simulink model "Utkarsh_2005574_R_W1_P3"  (R2021a)
settings: Solver=FixedStepDiscrete  StartTime=0.0  StopTime=0.1  RelTol=1e-3
settings Model: Creator=Utkarsh Anand  LastModifiedBy=Utkarsh Anand

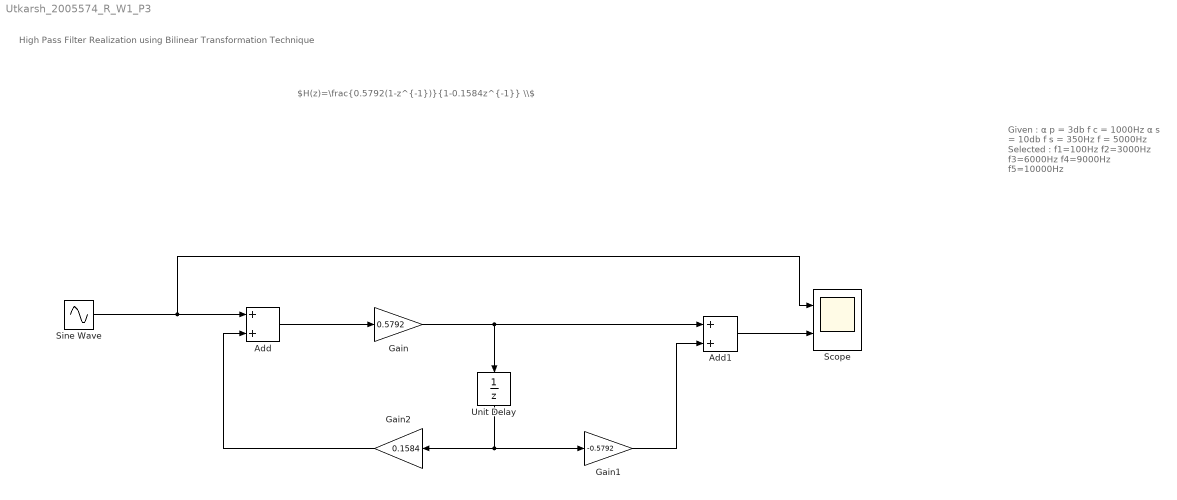
== system Utkarsh_2005574_R_W1_P3 ==
  note: $H(z)=\frac{0.5792(1-z^{-1})}{1-0.1584z^{-1}} \\$
  note: High Pass Filter Realization using Bilinear Transformation Technique
  note: Given :
      | α p = 3db
      | f c = 1000Hz
      | α s = 10db
      | f s = 350Hz
      | f = 5000Hz
      |
      | Selected :
      | f1=100Hz
      | f2=3000Hz
      | f3=6000Hz
      | f4=9000Hz
      | f5=10000Hz
  Add : Sum
  Add1 : Sum
  Gain : Gain  Gain=0.5792
  Gain1 : Gain  Gain=-0.5792
  Gain2 : Gain  Gain=0.1584
  Scope : Scope  NumInputPorts=2
  Sine Wave : Sin  Frequency=10000*2*pi  SampleTime=1/5000
  Unit Delay : UnitDelay  SampleTime=-1  HasFrameUpgradeWarning=on
  wires:
  Unit Delay/1 -> Gain2/1, Gain1/1
  Add/1 -> Gain/1
  Sine Wave/1 -> Scope/1, Add/1
  Add1/1 -> Scope/2
  Gain/1 -> Unit Delay/1, Add1/1
  Gain2/1 -> Add/2
  Gain1/1 -> Add1/2
